simulink model "drive1m_real"  (R2022a)
settings: Solver=FixedStepAuto  StartTime=0.0  StopTime=10.0  RelTol=1e-3  EnableMultiTasking=on
undefined symbols (not defined in the file): InputPWM, ticksPerRot, wheelR, WheelSpeed
libraries: arduinolib x10, spsEdgeDetectorLib x2, mobileRoboticsTrainingLib x1
settings Model: ExtModeTrigDuration=2  Creator=heath  LastModifiedBy=heath
settings OptimizationCC: EnhancedBackFolding=on  PassReuseOutputArgsAs=Individual arguments  ZeroExternalMemoryAtStartup=off  ZeroInternalMemoryAtStartup=off  MaxStackSize=64  OptimizeBlockOrder=speed  DifferentSizesBufferReuse=on  OptimizationCustomize=off  EfficientTunableParamExpr=on
settings DebuggingCC: MultiTaskDSMMsg=none  ParameterTunabilityLossMsg=error
settings HardwareCC: ProdBitPerPointer=32  ProdBitPerSizeT=32  ProdBitPerPtrDiffT=32  ProdLargestAtomicInteger=Long  ProdLargestAtomicFloat=Double  ProdWordSize=32  ProdHWDeviceType=ARM Compatible->ARM Cortex  UseEmbeddedCoderFeatures=off  UseSimulinkCoderFeatures=off
settings SFSimCC: MATLABDynamicMemAlloc=off
settings RTWCC: SystemTargetFile=ert.tlc  HardwareBoard=Arduino Nano 33 IoT  TemplateMakefile=ert_default_tmf  Toolchain=Arduino ARM  BuildConfiguration=Faster Runs
settings CodeAppCC: ForceParamTrailComments=on  IgnoreCustomStorageClasses=off  OperatorAnnotations=on  SimulinkDataObjDesc=on  SFDataObjDesc=on  InsertBlockDesc=on
settings ERTTargetCC: SupportContinuousTime=on  SupportNonInlinedSFcns=on  SupportVariableSizeSignals=on  ExtModeTransport=3  ExtModeStaticAlloc=on  ExtModeStaticAllocSize=8192  ExtModeMexFile=ext_xcp  ExtModeIntrfLevel=Level2 - Open

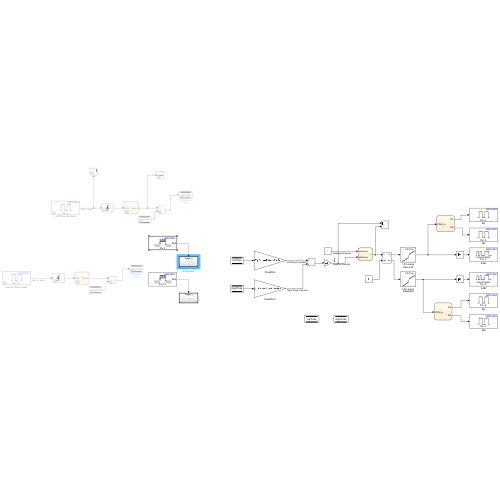
[thumbnail: Simulink's stored preview of the top-level diagram]
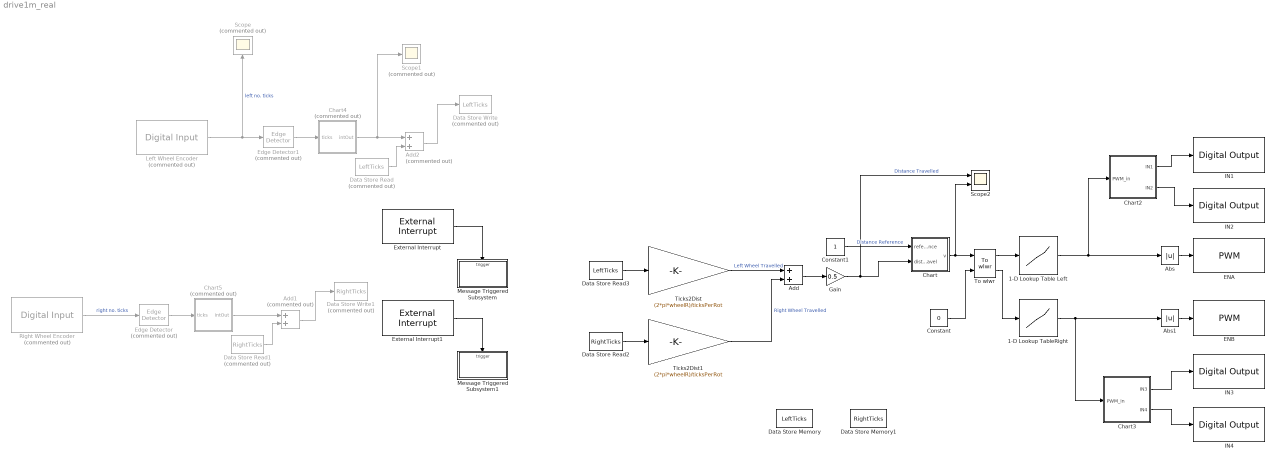
== system drive1m_real ==
  1-D Lookup Table Left : Lookup_n-D  NumberOfTableDimensions=1  BreakpointsForDimension1=WheelSpeed  Table=InputPWM  InternalRulePriority=Speed  RndMeth=Simplest
  1-D Lookup TableRight : Lookup_n-D  NumberOfTableDimensions=1  BreakpointsForDimension1=WheelSpeed  Table=InputPWM  InternalRulePriority=Speed  RndMeth=Simplest
  Abs : Abs  SaturateOnIntegerOverflow=off
  Abs1 : Abs  SaturateOnIntegerOverflow=off
  Add : Sum
  Add1 : Sum  Commented=on
  Add2 : Sum  Commented=on
  Chart : Stateflow chart  TreatAsAtomicUnit=on
  Chart2 : Stateflow chart  TreatAsAtomicUnit=on
  Chart3 : Stateflow chart  TreatAsAtomicUnit=on
  Chart4 : Stateflow chart  Commented=on  TreatAsAtomicUnit=on
  Chart5 : Stateflow chart  Commented=on  TreatAsAtomicUnit=on
  Constant : Constant  Value=0
  Constant1 : Constant
  Data Store Memory : DataStoreMemory  DataStoreName=LeftTicks  WriteAfterWriteMsg=warning  ShowAdditionalParam=off
  Data Store Memory1 : DataStoreMemory  DataStoreName=RightTicks  WriteAfterWriteMsg=warning  ShowAdditionalParam=off
  Data Store Read : DataStoreRead  Commented=on  DataStoreName=LeftTicks  IndexOptions=Index vector (dialog)  Indices=1  OutputSizes=1
  Data Store Read1 : DataStoreRead  Commented=on  DataStoreName=RightTicks  IndexOptions=Index vector (dialog)  Indices=1  OutputSizes=1
  Data Store Read2 : DataStoreRead  DataStoreName=RightTicks  IndexOptions=Index vector (dialog)  Indices=1  OutputSizes=1
  Data Store Read3 : DataStoreRead  DataStoreName=LeftTicks  IndexOptions=Index vector (dialog)  Indices=1  OutputSizes=1
  Data Store Write : DataStoreWrite  Commented=on  DataStoreName=LeftTicks  IndexOptions=Index vector (dialog)  Indices=1  OutputSizes=1
  Data Store Write1 : DataStoreWrite  Commented=on  DataStoreName=RightTicks  IndexOptions=Index vector (dialog)  Indices=1  OutputSizes=1
  ENA : arduinolib/PWM  pinNumber=3  frequencyType=Default  desiredFrequency=490.2  achievableFrequency=490.2
  ENB : arduinolib/PWM  pinNumber=2  frequencyType=Default  desiredFrequency=490.2  achievableFrequency=490.2
  Edge Detector : spsEdgeDetectorLib/Edge Detector  Commented=on  model=Rising  ic=0  Ts=0
      settings: SourceProductBaseCode=PS
  Edge Detector1 : spsEdgeDetectorLib/Edge Detector  Commented=on  model=Rising  ic=0  Ts=0
      settings: SourceProductBaseCode=PS
  External Interrupt : arduinolib/External Interrupt  Pin=9  PullUp=off  Mode=RISING  InterruptSimulationInput=off
      settings: SourceProductBaseCode=ARDUINO
  External Interrupt1 : arduinolib/External Interrupt  Pin=10  PullUp=off  Mode=RISING  InterruptSimulationInput=off
      settings: SourceProductBaseCode=ARDUINO
  Gain : Gain  Gain=0.5
  IN1 : arduinolib/Digital Output  pinNumber=4  Direction=output  blockPlatform=arduino
  IN2 : arduinolib/Digital Output  pinNumber=5  Direction=output  blockPlatform=arduino
  IN3 : arduinolib/Digital Output  pinNumber=6  Direction=output  blockPlatform=arduino
  IN4 : arduinolib/Digital Output  pinNumber=7  Direction=output  blockPlatform=arduino
  Left Wheel Encoder : arduinolib/Digital Input  Commented=on  pinNumber=9  mode=Default  Direction=input  SampleTime=0.1  blockPlatform=arduino
  Message Triggered Subsystem : Subsystem  TreatAsAtomicUnit=on
  Message Triggered Subsystem1 : Subsystem  TreatAsAtomicUnit=on
  Right Wheel Encoder : arduinolib/Digital Input  Commented=on  pinNumber=10  mode=Default  Direction=input  SampleTime=0.1  blockPlatform=arduino
  Scope : Scope  Commented=on
  Scope1 : Scope  Commented=on
  Scope2 : Scope  NumInputPorts=2
  Ticks2Dist : Gain  Gain=(2*pi*wheelR)/ticksPerRot
  Ticks2Dist1 : Gain  Gain=(2*pi*wheelR)/ticksPerRot
  To wlwr : mobileRoboticsTrainingLib/To wlwr  axleLength=axleLength  wheelR=wheelR
  wires:
  Chart/1(v) -> Scope2/2, To wlwr/1
  To wlwr/1 -> 1-D Lookup Table Left/1
  To wlwr/2 -> 1-D Lookup TableRight/1
  1-D Lookup TableRight/1 -> Chart3/1(PWM_in), Abs1/1
  Constant1/1 -> Chart/1(reference)  "Distance Reference"
  Ticks2Dist/1 -> Add/1  "Left Wheel Travelled"
  1-D Lookup Table Left/1 -> Chart2/1(PWM_in), Abs/1
  Constant/1 -> To wlwr/2
  Gain/1 -> Scope2/1, Chart/2(distTravel)  "Distance Travelled"
  Ticks2Dist1/1 -> Add/2  "Right Wheel Travelled"
  Add/1 -> Gain/1
  Left Wheel Encoder/1 -> Scope/1, Edge Detector1/1  "left no. ticks"
  Right Wheel Encoder/1 -> Edge Detector/1  "right no. ticks"
  Abs/1 -> ENA/1
  Abs1/1 -> ENB/1
  Chart2/1(IN1) -> IN1/1
  Chart2/2(IN2) -> IN2/1
  Chart3/1(IN3) -> IN3/1
  Chart3/2(IN4) -> IN4/1
  Edge Detector/1 -> Chart5/1(ticks)
  Edge Detector1/1 -> Chart4/1(ticks)
  Data Store Read1/1 -> Add1/2
  Chart4/1(intOut) -> Scope1/1, Add2/1
  Chart5/1(intOut) -> Add1/1
  Data Store Read/1 -> Add2/2
  Add1/1 -> Data Store Write1/1
  Add2/1 -> Data Store Write/1
  Data Store Read2/1 -> Ticks2Dist1/1
  Data Store Read3/1 -> Ticks2Dist/1
  External Interrupt/1 -> Message Triggered Subsystem/Trigger
  External Interrupt1/1 -> Message Triggered Subsystem1/Trigger

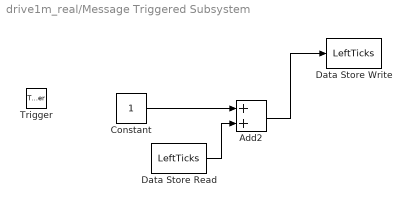
== system drive1m_real/Message Triggered Subsystem ==
  Trigger : TriggerPort  TriggerType=function-call  VariantControl=(inherit)  PortDimensions=1
  Add2 : Sum
  Constant : Constant
  Data Store Read : DataStoreRead  DataStoreName=LeftTicks  IndexOptions=Index vector (dialog)  Indices=1  OutputSizes=1
  Data Store Write : DataStoreWrite  DataStoreName=LeftTicks  IndexOptions=Index vector (dialog)  Indices=1  OutputSizes=1
  wires:
  Add2/1 -> Data Store Write/1
  Constant/1 -> Add2/1
  Data Store Read/1 -> Add2/2

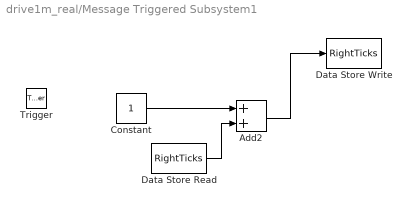
== system drive1m_real/Message Triggered Subsystem1 ==
  Trigger : TriggerPort  TriggerType=function-call  VariantControl=(inherit)  PortDimensions=1
  Add2 : Sum
  Constant : Constant
  Data Store Read : DataStoreRead  DataStoreName=RightTicks  IndexOptions=Index vector (dialog)  Indices=1  OutputSizes=1
  Data Store Write : DataStoreWrite  DataStoreName=RightTicks  IndexOptions=Index vector (dialog)  Indices=1  OutputSizes=1
  wires:
  Add2/1 -> Data Store Write/1
  Constant/1 -> Add2/1
  Data Store Read/1 -> Add2/2

== stateflow chart drive1m_real/Chart2 ==
  state Forward
    entry:
    IN1 = 1;
    IN2 = 0;
  state Back
    entry:
    IN1 = 0;
    IN2 = 1;
  (default) -> Forward
  Forward -> Back : [PWM_in<0]
  Back -> Forward : [PWM_in>=0]
  data: PWM_in input; IN1 output; IN2 output

== stateflow chart drive1m_real/Chart ==
  state MoveForward
    entry:
    v = 0.2;
  state Stop
    entry:
    v = 0;
  (default) -> MoveForward
  MoveForward -> Stop : [distTravel > reference]
  data: reference input; distTravel input; v output

== stateflow chart drive1m_real/Chart3 ==
  state Forward
    entry:
    IN4 = 0;
    IN3 = 1;
  state Back
    entry:
    IN4 = 1;
    IN3 = 0;
  (default) -> Forward
  Forward -> Back : [PWM_in<0]
  Back -> Forward : [PWM_in>=0]
  data: PWM_in input; IN3 output; IN4 output

== stateflow chart drive1m_real/Chart4 ==
  (default) -> (junction 10) : % GetIfTick
      | {intOut = 0}
  (junction 10) -> (junction 11) [order 1] : [ticks]
  (junction 10) -> (junction 12) [order 2] : {intOut = 0;}
  (junction 11) -> (junction 13) : {intOut = 1;}
  (junction 13) -> (junction 12)
  (junction 12) -> (junction 14)
  data: ticks input; intOut output

== stateflow chart drive1m_real/Chart5 ==
  (default) -> (junction 10) : % GetIfTick
  (junction 10) -> (junction 11) [order 1] : [ticks > 0]
  (junction 10) -> (junction 12) [order 2] : {intOut = 0;}
  (junction 11) -> (junction 13) : {intOut = 1;}
  (junction 13) -> (junction 12)
  (junction 12) -> (junction 14)
  data: ticks input; intOut output
